simulink subsystem "s0506_th_ddot_pid"  (R2019b)
settings: Solver=VariableStepAuto  StartTime=0.0  StopTime=10.0  RelTol=1e-3
undefined symbols (not defined in the file): __PRM__SERIALIZED__DATA__, PARAMS, SubsystemReferenceBlock
settings Model: Creator=alessandro  LastModifiedBy=alessandro

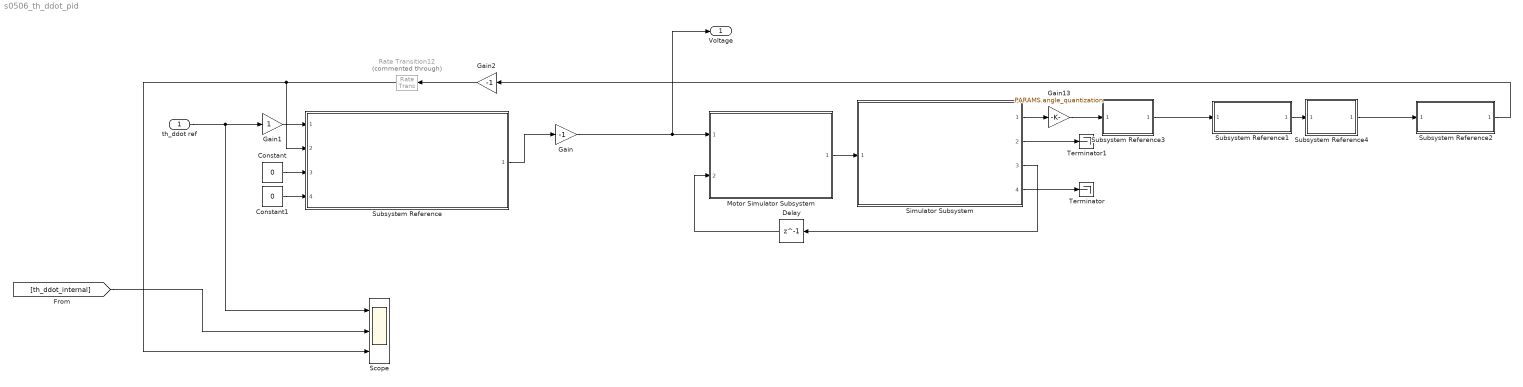
== system s0506_th_ddot_pid ==
  th_ddot ref : Inport
  Constant : Constant  Value=0
  Constant1 : Constant  Value=0
  Delay : Delay  DelayLength=1
  Gain : Gain  Gain=-1
  Gain1 : Gain
  Gain13 : Gain  Gain=PARAMS.angle_quantization
  Gain2 : Gain  Gain=-1
  Motor Simulator Subsystem : Subsystem  ReferencedSubsystem=s0303_motor_simulator  omega_0=PARAMS.th_dot_0  i_0=0
  Rate Transition12 : RateTransition  Commented=through  OutPortSampleTime=dt_control
  Scope : Scope  NumInputPorts=3
  Simulator Subsystem : Subsystem  ReferencedSubsystem=s0323_mechanical_simulator2  th_0=PARAMS.th_0  al_0=PARAMS.al_0  th_dot_0=PARAMS.th_dot_0  al_dot_0=PARAMS.al_dot_0
  Subsystem Reference : Subsystem  BlockKeywords=__PRM__SERIALIZED__DATA__:SubsystemReferenceBlock  ReferencedSubsystem=s0307_theta_controller_PID  wc=20  cz_ratio=10  pc_ratio=10
  Subsystem Reference1 : Subsystem  BlockKeywords=__PRM__SERIALIZED__DATA__:SubsystemReferenceBlock  ReferencedSubsystem=Filtered_Derivative  num=num_der_filter  den=den_der_filter
  Subsystem Reference2 : Subsystem  BlockKeywords=__PRM__SERIALIZED__DATA__:SubsystemReferenceBlock  ReferencedSubsystem=Filtered_Derivative  num=num_der_filter  den=den_der_filter
  Subsystem Reference3 : Subsystem  BlockKeywords=__PRM__SERIALIZED__DATA__:SubsystemReferenceBlock  ReferencedSubsystem=Polynomial_Filter
  Subsystem Reference4 : Subsystem  BlockKeywords=__PRM__SERIALIZED__DATA__:SubsystemReferenceBlock  ReferencedSubsystem=Polynomial_Filter
  Terminator : Terminator
  Terminator1 : Terminator
  Voltage : Outport
  wires:
  Motor Simulator Subsystem/1 -> Simulator Subsystem/1
  Simulator Subsystem/3 -> Delay/1
  Simulator Subsystem/1 -> Gain13/1
  Simulator Subsystem/2 -> Terminator1/1
  Simulator Subsystem/4 -> Terminator/1
  Subsystem Reference/1 -> Gain/1
  th_ddot ref/1 -> Gain1/1, Scope/1
  Constant/1 -> Subsystem Reference/3
  Constant1/1 -> Subsystem Reference/4
  Delay/1 -> Motor Simulator Subsystem/2
  Gain/1 -> Motor Simulator Subsystem/1, Voltage/1
  Subsystem Reference3/1 -> Subsystem Reference1/1
  Subsystem Reference4/1 -> Subsystem Reference2/1
  Subsystem Reference1/1 -> Subsystem Reference4/1
  Subsystem Reference2/1 -> Gain2/1
  [th_ddot_internal] -> Scope/2
  Gain1/1 -> Subsystem Reference/1
  Gain13/1 -> Subsystem Reference3/1
  Rate Transition12/1 -> Scope/3, Subsystem Reference/2
  Gain2/1 -> Rate Transition12/1
